simulink model "SWC_DID_type"  (R2021b)
settings: Solver=FixedStepDiscrete  StartTime=0.0  StopTime=10.0  RelTol=1e-3
(part 2 of 2)

== system SWC_DID_type/P_DIDWriteCDD/run_DIDSet_UWBAnchorSta_sys ==
  note: Added blocks
  note: Added blocks
  note: Added blocks
  note: Added blocks
  function : TriggerPort  TriggerType=function-call  IsSimulinkFunction=on  FunctionName=run_DIDSet_UWBAnchorSta  VariantControl=(inherit)
  Terminator_1 : Terminator
  Terminator_2 : Terminator
  Terminator_3 : Terminator
  u16_DIDNum_UWBAnchorSta : ArgIn  OutDataTypeStr=uint16  ArgumentName=u16_DIDNum_UWBAnchorSta
  u16_DIDLen_UWBAnchorSta : ArgIn  Port=2  OutDataTypeStr=uint16  ArgumentName=u16_DIDLen_UWBAnchorSta
  u8Array93_UWBAnchorSta : ArgIn  Port=3  OutDataTypeStr=uint8  PortDimensions=93  ArgumentName=u8Array93_UWBAnchorSta
  wires:
  u16_DIDNum_UWBAnchorSta/1 -> Terminator_1/1
  u16_DIDLen_UWBAnchorSta/1 -> Terminator_2/1
  u8Array93_UWBAnchorSta/1 -> Terminator_3/1

== system SWC_DID_type/P_DIDWriteCDD/run_DIDSet_VIN_sys ==
  note: Added blocks
  note: Added blocks
  note: Added blocks
  note: Added blocks
  function : TriggerPort  TriggerType=function-call  IsSimulinkFunction=on  FunctionName=run_DIDSet_VIN  VariantControl=(inherit)
  Terminator_1 : Terminator
  Terminator_2 : Terminator
  Terminator_3 : Terminator
  u16_DIDNum_VIN : ArgIn  OutDataTypeStr=uint16  ArgumentName=u16_DIDNum_VIN
  u16_DIDLen_VIN : ArgIn  Port=2  OutDataTypeStr=uint16  ArgumentName=u16_DIDLen_VIN
  u8Array17_VIN : ArgIn  Port=3  OutDataTypeStr=uint8  PortDimensions=17  ArgumentName=u8Array17_VIN
  wires:
  u16_DIDNum_VIN/1 -> Terminator_1/1
  u16_DIDLen_VIN/1 -> Terminator_2/1
  u8Array17_VIN/1 -> Terminator_3/1

== system SWC_DID_type/P_DIDWriteCDD/run_DIDSet_VSS_sys ==
  note: Added blocks
  note: Added blocks
  note: Added blocks
  note: Added blocks
  function : TriggerPort  TriggerType=function-call  IsSimulinkFunction=on  FunctionName=run_DIDSet_VSS  VariantControl=(inherit)
  Terminator_1 : Terminator
  Terminator_2 : Terminator
  Terminator_3 : Terminator
  u16_DIDNum_VSS : ArgIn  OutDataTypeStr=uint16  ArgumentName=u16_DIDNum_VSS
  u16_DIDLen_VSS : ArgIn  Port=2  OutDataTypeStr=uint16  ArgumentName=u16_DIDLen_VSS
  u8_VSS : ArgIn  Port=3  OutDataTypeStr=uint8  ArgumentName=u8_VSS
  wires:
  u16_DIDNum_VSS/1 -> Terminator_1/1
  u16_DIDLen_VSS/1 -> Terminator_2/1
  u8_VSS/1 -> Terminator_3/1

== system SWC_DID_type/P_DIDWriteCDD/run_DIDSet_WhlPres_sys ==
  function : TriggerPort  TriggerType=function-call  IsSimulinkFunction=on  FunctionName=run_DIDSet_WhlPres  VariantControl=(inherit)
  Terminator_1 : Terminator
  Terminator_2 : Terminator
  Terminator_3 : Terminator
  u16_DIDNum_WhlPres : ArgIn  OutDataTypeStr=uint16  ArgumentName=u16_DIDNum_WhlPres
  u16_DIDLen_WhlPres : ArgIn  Port=2  OutDataTypeStr=uint16  ArgumentName=u16_DIDLen_WhlPres
  u8Array4_WhlPres : ArgIn  Port=3  OutDataTypeStr=uint8  PortDimensions=4  ArgumentName=u8Array4_WhlPres
  wires:
  u16_DIDNum_WhlPres/1 -> Terminator_1/1
  u16_DIDLen_WhlPres/1 -> Terminator_2/1
  u8Array4_WhlPres/1 -> Terminator_3/1

== system SWC_DID_type/P_DIDWriteCDD/run_DIDSet_WhlSensorBattSta_sys ==
  function : TriggerPort  TriggerType=function-call  IsSimulinkFunction=on  FunctionName=run_DIDSet_WhlSensorBattSta  VariantControl=(inherit)
  Terminator_1 : Terminator
  Terminator_2 : Terminator
  Terminator_3 : Terminator
  u16_DIDNum_WhlSensorBattSta : ArgIn  OutDataTypeStr=uint16  ArgumentName=u16_DIDNum_WhlSensorBattSta
  u16_DIDLen_WhlSensorBattSta : ArgIn  Port=2  OutDataTypeStr=uint16  ArgumentName=u16_DIDLen_WhlSensorBattSta
  u8_WhlSensorBattSta : ArgIn  Port=3  OutDataTypeStr=uint8  ArgumentName=u8_WhlSensorBattSta
  wires:
  u16_DIDNum_WhlSensorBattSta/1 -> Terminator_1/1
  u16_DIDLen_WhlSensorBattSta/1 -> Terminator_2/1
  u8_WhlSensorBattSta/1 -> Terminator_3/1

== system SWC_DID_type/P_DIDWriteCDD/run_DIDSet_WhlTmp_sys ==
  function : TriggerPort  TriggerType=function-call  IsSimulinkFunction=on  FunctionName=run_DIDSet_WhlTmp  VariantControl=(inherit)
  Terminator_1 : Terminator
  Terminator_2 : Terminator
  Terminator_3 : Terminator
  u16_DIDNum_WhlTmp : ArgIn  OutDataTypeStr=uint16  ArgumentName=u16_DIDNum_WhlTmp
  u16_DIDLen_WhlTmp : ArgIn  Port=2  OutDataTypeStr=uint16  ArgumentName=u16_DIDLen_WhlTmp
  u8Array4_WhlTmp : ArgIn  Port=3  OutDataTypeStr=uint8  PortDimensions=4  ArgumentName=u8Array4_WhlTmp
  wires:
  u16_DIDNum_WhlTmp/1 -> Terminator_1/1
  u16_DIDLen_WhlTmp/1 -> Terminator_2/1
  u8Array4_WhlTmp/1 -> Terminator_3/1

== system SWC_DID_type/P_DIDWriteCDD/run_DIDSet_WipRLSCmdCutFilter_sys ==
  function : TriggerPort  TriggerType=function-call  IsSimulinkFunction=on  FunctionName=run_DIDSet_WipRLSCmdCutFilter  VariantControl=(inherit)
  Terminator_1 : Terminator
  Terminator_2 : Terminator
  Terminator_3 : Terminator
  u16_DIDNum_WipRLSCmdCutFilter : ArgIn  OutDataTypeStr=uint16  ArgumentName=u16_DIDNum_WipRLSCmdCutFilter
  u16_DIDLen_WipRLSCmdCutFilter : ArgIn  Port=2  OutDataTypeStr=uint16  ArgumentName=u16_DIDLen_WipRLSCmdCutFilter
  u8_WipRLSCmdCutFilter : ArgIn  Port=3  OutDataTypeStr=uint8  ArgumentName=u8_WipRLSCmdCutFilter
  wires:
  u16_DIDNum_WipRLSCmdCutFilter/1 -> Terminator_1/1
  u16_DIDLen_WipRLSCmdCutFilter/1 -> Terminator_2/1
  u8_WipRLSCmdCutFilter/1 -> Terminator_3/1

== system SWC_DID_type/P_DIDWriteCDD/run_DIDSet_WipRLSCmdHoldFilter_sys ==
  function : TriggerPort  TriggerType=function-call  IsSimulinkFunction=on  FunctionName=run_DIDSet_WipRLSCmdHoldFilter  VariantControl=(inherit)
  Terminator_1 : Terminator
  Terminator_2 : Terminator
  Terminator_3 : Terminator
  u16_DIDNum_WipRLSCmdHoldFilter : ArgIn  OutDataTypeStr=uint16  ArgumentName=u16_DIDNum_WipRLSCmdHoldFilter
  u16_DIDLen_WipRLSCmdHoldFilter : ArgIn  Port=2  OutDataTypeStr=uint16  ArgumentName=u16_DIDLen_WipRLSCmdHoldFilter
  u8_WipRLSCmdHoldFilter : ArgIn  Port=3  OutDataTypeStr=uint8  ArgumentName=u8_WipRLSCmdHoldFilter
  wires:
  u16_DIDNum_WipRLSCmdHoldFilter/1 -> Terminator_1/1
  u16_DIDLen_WipRLSCmdHoldFilter/1 -> Terminator_2/1
  u8_WipRLSCmdHoldFilter/1 -> Terminator_3/1

== system SWC_DID_type/P_DIDWriteCDD/run_DIDSet_XWDMode_sys ==
  function : TriggerPort  TriggerType=function-call  IsSimulinkFunction=on  FunctionName=run_DIDSet_XWDMode  VariantControl=(inherit)
  Terminator_1 : Terminator
  Terminator_2 : Terminator
  Terminator_3 : Terminator
  u16_DIDNum_XWDMode : ArgIn  OutDataTypeStr=uint16  ArgumentName=u16_DIDNum_XWDMode
  u16_DIDLen_XWDMode : ArgIn  Port=2  OutDataTypeStr=uint16  ArgumentName=u16_DIDLen_XWDMode
  u8_XWDMode : ArgIn  Port=3  OutDataTypeStr=uint8  ArgumentName=u8_XWDMode
  wires:
  u16_DIDNum_XWDMode/1 -> Terminator_1/1
  u16_DIDLen_XWDMode/1 -> Terminator_2/1
  u8_XWDMode/1 -> Terminator_3/1
